simulink model "Practica4_simulink"  (R2023a)
settings: Solver=ode23  StartTime=0.0  StopTime=15  RelTol=1e-3
values from neighbouring files (symbols this model uses):
  k = 100    [P4_MovRyT.m]
  m = 10    [P4_MovRyT.m]
  r = 0.05    [P4_MovRyT.m]
settings Model: Creator=karen  LastModifiedBy=karen

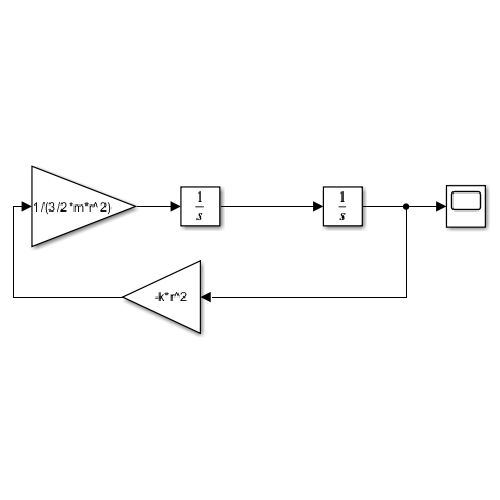
[thumbnail: Simulink's stored preview of the top-level diagram]
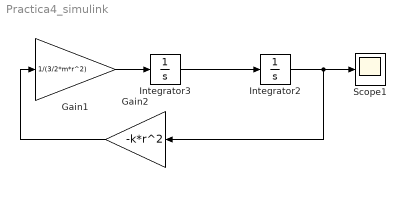
== system Practica4_simulink ==
  Gain1 : Gain  Gain=1/(3/2*m*r^2)
  Gain2 : Gain  Gain=-k*r^2
  Integrator2 : Integrator
  Integrator3 : Integrator  InitialCondition=2
  Scope1 : Scope
  wires:
  Integrator2/1 -> Gain2/1, Scope1/1
  Integrator3/1 -> Integrator2/1
  Gain1/1 -> Integrator3/1
  Gain2/1 -> Gain1/1
